simulink model "bus_test"  (Simulink 8.4)
settings: Solver=VariableStepDiscrete  StartTime=0.0  StopTime=0  MaxStep=1  RelTol=1e-3
undefined symbols (not defined in the file or in its folder): BusA_MATLABStruct
settings Model: Creator=arnaud  LastModifiedBy=arnaud
settings DataIOCC: SaveFormat=Structure  SignalLoggingSaveFormat=Dataset
settings OptimizationCC: ExpressionDepthLimit=128
settings DebuggingCC: UnderspecifiedInitializationDetection=Simplified  MergeDetectMultiDrivingBlocksExec=error  FcnCallInpInsideContextMsg=EnableAllAsError  StateNameClashWarn=none
settings GRTTargetCC: CombineOutputUpdateFcns=on  GRTInterface=off

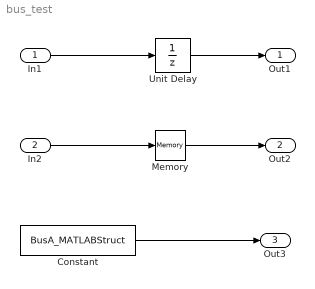
== system bus_test ==
  In1 : Inport  OutDataTypeStr=Bus: BusA  BusOutputAsStruct=on
  In2 : Inport  Port=2  OutDataTypeStr=Bus: BusB  BusOutputAsStruct=on
  Constant : Constant  Value=BusA_MATLABStruct  OutDataTypeStr=Bus: BusA
  Memory : Memory
  Unit Delay : UnitDelay  InitialCondition=1  SampleTime=-1
  Out1 : Outport
  Out2 : Outport  Port=2
  Out3 : Outport  Port=3
  wires:
  In1/1 -> Unit Delay/1
  In2/1 -> Memory/1
  Unit Delay/1 -> Out1/1
  Memory/1 -> Out2/1
  Constant/1 -> Out3/1
